simulink model "simulation_model_3"  (R2022b)
settings: Solver=ode3  StartTime=0.0  StopTime=Tsim  FixedStep=DTsim  RelTol=1e-3  EnableMultiTasking=on
values from neighbouring files (symbols this model uses):
  d1_step_final_value = 10    [simulation_script.m]
  d1_step_initial_value = 0    [simulation_script.m]
  d1_step_start = 5    [simulation_script.m]
  d1_step_stop = Tsim+1    (= 101)    [simulation_script.m]
  d2_step_final_value = 5    [simulation_script.m]
  d2_step_initial_value = 0    [simulation_script.m]
  d2_step_start = 10    [simulation_script.m]
  d2_step_stop = Tsim+1    (= 101)    [simulation_script.m]
  f = 0.1    [simulation_script.m]
  g = 9.81    [simulation_script.m]
  J = 0.2    [simulation_script.m]
  kd_gx = 2*omega*epsilon    (= 8)    [simulation_script.m]
  kd_gz = 2*omega*epsilon    (= 8)    [simulation_script.m]
  kp_gx = omega^2    (= 32.6530612245)    [simulation_script.m]
  kp_gz = omega^2    (= 32.6530612245)    [simulation_script.m]
  Lmax = 200    [simulation_script.m]
  Lmin = 0    [simulation_script.m]
  m = 10    [simulation_script.m]
  tau = 0.1    [simulation_script.m]
  Tmax = 0.035    [simulation_script.m]
  Tmin = -0.035    [simulation_script.m]
settings Model: Creator=mouyon  LastModifiedBy=Akash
settings SolverCC: AlgebraicLoopSolver=TrustRegion
settings DataIOCC: LimitDataPoints=on  SaveFormat=Array  SignalLoggingSaveFormat=ModelDataLogs  ReturnWorkspaceOutputs=off
settings OptimizationCC: ExpressionDepthLimit=2147483647  InitFltsAndDblsToZero=on  LifeSpan=inf
settings DebuggingCC: UnderspecifiedInitializationDetection=Classic  MergeDetectMultiDrivingBlocksExec=none  SolverPrmCheckMsg=warning  FcnCallInpInsideContextMsg=warning  UnconnectedInputMsg=warning  UnconnectedOutputMsg=warning  UnconnectedLineMsg=warning  AllowSymbolicDim=off  StateNameClashWarn=warning  SFUnexpectedBacktrackingDiag=warning  SFNoUnconditionalDefaultTransitionDiag=warning  SFExecutionAtInitializationDiag=none  SFMachineParentedDataDiag=warning  ArithmeticOperatorsInVariantConditions=warning
settings HardwareCC: ProdBitPerPointer=32  ProdBitPerSizeT=32  ProdBitPerPtrDiffT=32  ProdLargestAtomicFloat=None  ProdIntDivRoundTo=Undefined  ProdEndianess=Unspecified  ProdWordSize=32  ProdHWDeviceType=32-bit Generic
settings ModelReferenceCC: EnableRefExpFcnMdlSchedulingChecks=on  PropagateSignalLabelsOutOfModel=off
settings SFSimCC: SimUseLocalCustomCode=off  CustomCodeUndefinedFunction=UseInterfaceOnly
settings RTWCC: RTWUseLocalCustomCode=off
settings CodeAppCC: StateflowObjectComments=on
settings GRTTargetCC: TargetLangStandard=C89/C90 (ANSI)  CombineOutputUpdateFcns=off  GRTInterface=on
settings ConfigComp: CovMetricSettings=dw  CovSaveCumulativeToWorkspaceVar=on  CovSaveSingleToWorkspaceVar=on  CovExternalEMLEnable=off

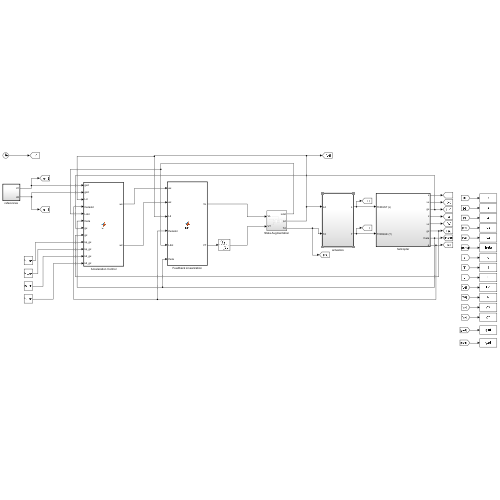
[thumbnail: Simulink's stored preview of the top-level diagram]
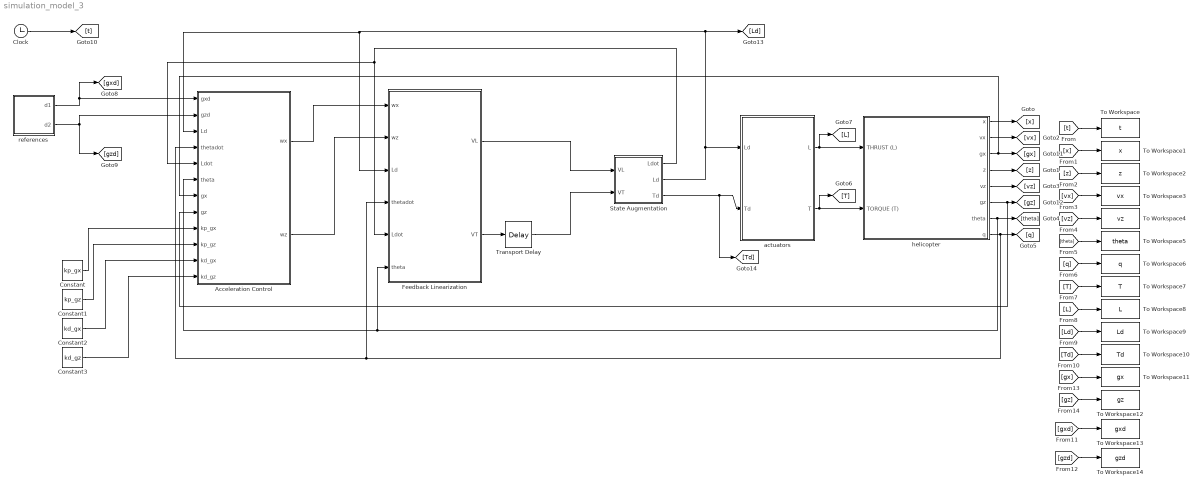
== system simulation_model_3 ==
  Acceleration Control : MATLAB Function  TreatAsAtomicUnit=on
  Clock : Clock
  Constant : Constant  Value=kp_gx
  Constant1 : Constant  Value=kp_gz
  Constant2 : Constant  Value=kd_gx
  Constant3 : Constant  Value=kd_gz
  Feedback Linearization : MATLAB Function  TreatAsAtomicUnit=on
  State Augmentation : Subsystem
  To Workspace : ToWorkspace  VariableName=t  SampleTime=-1
  To Workspace1 : ToWorkspace  VariableName=x  SampleTime=-1
  To Workspace10 : ToWorkspace  VariableName=Td  SampleTime=-1
  To Workspace11 : ToWorkspace  VariableName=gx  SampleTime=-1
  To Workspace12 : ToWorkspace  VariableName=gz  SampleTime=-1
  To Workspace13 : ToWorkspace  VariableName=gxd  SampleTime=-1
  To Workspace14 : ToWorkspace  VariableName=gzd  SampleTime=-1
  To Workspace2 : ToWorkspace  VariableName=z  SampleTime=-1
  To Workspace3 : ToWorkspace  VariableName=vx  SampleTime=-1
  To Workspace4 : ToWorkspace  VariableName=vz  SampleTime=-1
  To Workspace5 : ToWorkspace  VariableName=theta  SampleTime=-1
  To Workspace6 : ToWorkspace  VariableName=q  SampleTime=-1
  To Workspace7 : ToWorkspace  VariableName=T  SampleTime=-1
  To Workspace8 : ToWorkspace  VariableName=L  SampleTime=-1
  To Workspace9 : ToWorkspace  VariableName=Ld  SampleTime=-1
  Transport Delay : TransportDelay  DelayTime=0
  actuators : Subsystem  TreatAsAtomicUnit=on
  helicopter : Subsystem  TreatAsAtomicUnit=on
  references : Subsystem  TreatAsAtomicUnit=on
  wires:
  helicopter/1(x) -> [x]
  helicopter/5(vz) -> [vz]
  helicopter/7(theta) -> Feedback Linearization/6(theta), Acceleration Control/6(theta), [theta]
  helicopter/8(q) -> Acceleration Control/4(thetadot), Feedback Linearization/4(thetadot), [q]
  Clock/1 -> [t]
  [t] -> To Workspace/1
  [x] -> To Workspace1/1
  [z] -> To Workspace2/1
  [vx] -> To Workspace3/1
  [vz] -> To Workspace4/1
  [theta] -> To Workspace5/1
  [q] -> To Workspace6/1
  [T] -> To Workspace7/1
  [L] -> To Workspace8/1
  [Ld] -> To Workspace9/1
  [Td] -> To Workspace10/1
  helicopter/2(vx) -> [vx]
  helicopter/4(z) -> [z]
  helicopter/3(gx) -> Acceleration Control/7(gx), [gx]
  helicopter/6(gz) -> Acceleration Control/8(gz), [gz]
  [gx] -> To Workspace11/1
  [gz] -> To Workspace12/1
  actuators/1(L) -> helicopter/1(THRUST (L)), [L]
  actuators/2(T) -> helicopter/2(TORQUE (T)), [T]
  references/2(d2) -> [gzd], Acceleration Control/2(gzd)
  [gxd] -> To Workspace13/1
  [gzd] -> To Workspace14/1
  Feedback Linearization/2(VT) -> Transport Delay/1
  references/1(d1) -> [gxd], Acceleration Control/1(gxd)
  Acceleration Control/1(wx) -> Feedback Linearization/1(wx)
  Acceleration Control/2(wz) -> Feedback Linearization/2(wz)
  State Augmentation/1(Ldot) -> Feedback Linearization/5(Ldot), Acceleration Control/5(Ldot)
  State Augmentation/2(Ld) -> Acceleration Control/3(Ld), Feedback Linearization/3(Ld), [Ld], actuators/1(Ld)
  State Augmentation/3(Td) -> [Td], actuators/2(Td)
  Feedback Linearization/1(VL) -> State Augmentation/1(VL)
  Transport Delay/1 -> State Augmentation/2(VT)
  Constant/1 -> Acceleration Control/9(kp_gx)
  Constant1/1 -> Acceleration Control/10(kp_gz)
  Constant3/1 -> Acceleration Control/12(kd_gz)
  Constant2/1 -> Acceleration Control/11(kd_gx)

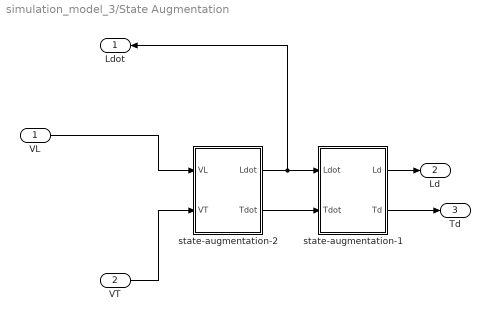
== system simulation_model_3/State Augmentation ==
  VL : Inport
  VT : Inport  Port=2
  state-augmentation-1 : Subsystem  TreatAsAtomicUnit=on
  state-augmentation-2 : Subsystem  TreatAsAtomicUnit=on
  Ldot : Outport
  Ld : Outport  Port=2
  Td : Outport  Port=3
  wires:
  state-augmentation-2/2(Tdot) -> state-augmentation-1/2(Tdot)
  state-augmentation-2/1(Ldot) -> Ldot/1, state-augmentation-1/1(Ldot)
  state-augmentation-1/1(Ld) -> Ld/1
  state-augmentation-1/2(Td) -> Td/1
  VL/1 -> state-augmentation-2/1(VL)
  VT/1 -> state-augmentation-2/2(VT)

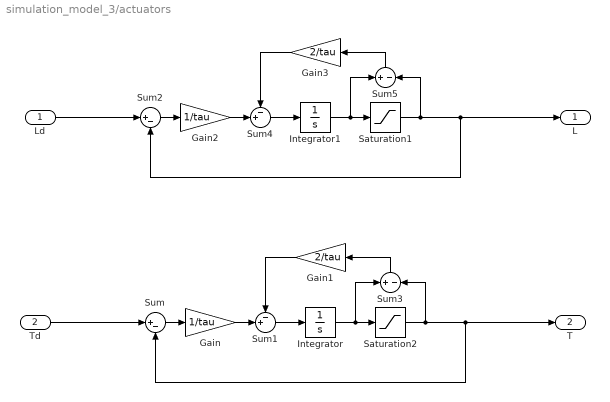
== system simulation_model_3/actuators ==
  Ld : Inport
  Td : Inport  Port=2
  Gain : Gain  Gain=1/tau
  Gain1 : Gain  Gain=2/tau
  Gain2 : Gain  Gain=1/tau
  Gain3 : Gain  Gain=2/tau
  Integrator : Integrator
  Integrator1 : Integrator  InitialCondition=m*g
  Saturation1 : Saturate  UpperLimit=Lmax  LowerLimit=Lmin
  Saturation2 : Saturate  UpperLimit=Tmax  LowerLimit=Tmin
  Sum : Sum  Inputs=|+-
  Sum1 : Sum  Inputs=-+|
  Sum2 : Sum  Inputs=|+-
  Sum3 : Sum  Inputs=+|-  SaturateOnIntegerOverflow=on
  Sum4 : Sum  Inputs=-+|
  Sum5 : Sum  Inputs=+|-  SaturateOnIntegerOverflow=on
  L : Outport
  T : Outport  Port=2
  wires:
  Integrator/1 -> Sum3/1, Saturation2/1
  Sum/1 -> Gain/1
  Td/1 -> Sum/1
  Sum3/1 -> Gain1/1
  Gain/1 -> Sum1/2
  Sum1/1 -> Integrator/1
  Integrator1/1 -> Saturation1/1, Sum5/1
  Sum2/1 -> Gain2/1
  Ld/1 -> Sum2/1
  Saturation1/1 -> Sum2/2, L/1, Sum5/2
  Sum5/1 -> Gain3/1
  Gain2/1 -> Sum4/2
  Sum4/1 -> Integrator1/1
  Gain3/1 -> Sum4/1
  Gain1/1 -> Sum1/1
  Saturation2/1 -> Sum/2, T/1, Sum3/2

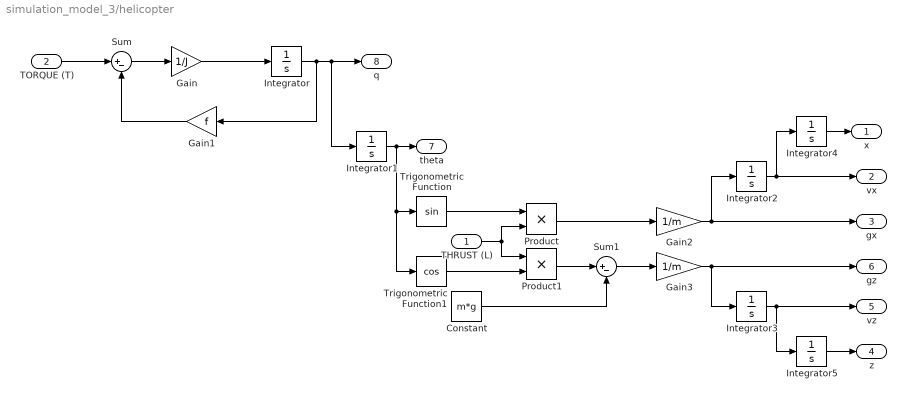
== system simulation_model_3/helicopter ==
  THRUST (L) : Inport
  TORQUE (T) : Inport  Port=2
  Constant : Constant  Value=m*g
  Gain : Gain  Gain=1/J
  Gain1 : Gain  Gain=f
  Gain2 : Gain  Gain=1/m
  Gain3 : Gain  Gain=1/m
  Integrator{,1..5} (6 alike) : Integrator
  Product : Product  RndMeth=Zero
  Product1 : Product  RndMeth=Zero
  Sum : Sum  Inputs=|+-
  Sum1 : Sum  Inputs=|+-
  Trigonometric Function : Trigonometry
  Trigonometric Function1 : Trigonometry  Operator=cos
  x : Outport
  vx : Outport  Port=2
  gx : Outport  Port=3
  z : Outport  Port=4
  vz : Outport  Port=5
  gz : Outport  Port=6
  theta : Outport  Port=7
  q : Outport  Port=8
  wires:
  Integrator/1 -> Gain1/1, q/1, Integrator1/1
  Gain/1 -> Integrator/1
  Gain1/1 -> Sum/2
  Sum/1 -> Gain/1
  TORQUE (T)/1 -> Sum/1
  Integrator1/1 -> theta/1, Trigonometric Function/1, Trigonometric Function1/1
  Trigonometric Function/1 -> Product/1
  THRUST (L)/1 -> Product/2, Product1/1
  Trigonometric Function1/1 -> Product1/2
  Product/1 -> Gain2/1
  Product1/1 -> Sum1/1
  Constant/1 -> Sum1/2
  Gain3/1 -> gz/1, Integrator3/1
  Sum1/1 -> Gain3/1
  Integrator2/1 -> vx/1, Integrator4/1
  Integrator3/1 -> vz/1, Integrator5/1
  Integrator4/1 -> x/1
  Integrator5/1 -> z/1
  Gain2/1 -> gx/1, Integrator2/1

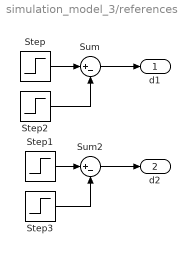
== system simulation_model_3/references ==
  Step : Step  Time=d1_step_start  Before=d1_step_initial_value  After=d1_step_final_value  SampleTime=0
  Step1 : Step  Time=d2_step_start  Before=d2_step_initial_value  After=d2_step_final_value  SampleTime=0
  Step2 : Step  Time=d1_step_stop  After=d1_step_final_value  SampleTime=0
  Step3 : Step  Time=d2_step_stop  After=d2_step_final_value  SampleTime=0
  Sum : Sum  Inputs=|+-
  Sum2 : Sum  Inputs=|+-
  d1 : Outport
  d2 : Outport  Port=2
  wires:
  Step/1 -> Sum/1
  Step2/1 -> Sum/2
  Step1/1 -> Sum2/1
  Sum/1 -> d1/1
  Sum2/1 -> d2/1
  Step3/1 -> Sum2/2

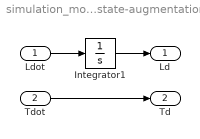
== system simulation_model_3/State Augmentation/state-augmentation-1 ==
  Ldot : Inport
  Tdot : Inport  Port=2
  Integrator1 : Integrator  InitialCondition=m*g
  Ld : Outport
  Td : Outport  Port=2
  wires:
  Integrator1/1 -> Ld/1
  Ldot/1 -> Integrator1/1
  Tdot/1 -> Td/1

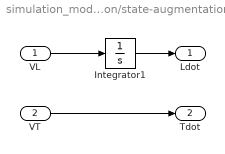
== system simulation_model_3/State Augmentation/state-augmentation-2 ==
  VL : Inport
  VT : Inport  Port=2
  Integrator1 : Integrator
  Ldot : Outport
  Tdot : Outport  Port=2
  wires:
  Integrator1/1 -> Ldot/1
  VL/1 -> Integrator1/1
  VT/1 -> Tdot/1

== matlab function simulation_model_3/Feedback Linearization ==
  data: wx input; VL output; wz input; VT output; Ld input; thetadot input; Ldot input; theta input
function [VL,VT] = fcn(wx, wz, Ld, thetadot, Ldot, theta)

m = 10;
J = 0.2;
f = 0.1;

A1 = [Ld*thetadot^2;
(thetadot*(Ld*f - 2*J*Ldot))/Ld];

A2 = [m*sin(theta)        m*cos(theta);
(J*m*cos(theta))/Ld -(J*m*sin(theta))/Ld];

Answer = A1 + A2*[wx;wz];
VL = Answer(1);
VT = Answer(2);
end

== matlab function simulation_model_3/Acceleration Control ==
  data: gxd input; wx output; gzd input; wz output; Ld input; thetadot input; Ldot input; theta input; gx input; gz input; kp_gx input; kp_gz input; kd_gx input; kd_gz input
function [wx,wz]  = fcn(gxd, gzd, Ld, thetadot, Ldot, theta, gx, gz, kp_gx, kp_gz, kd_gx, kd_gz)

m = 10;
%alpha1 = 8.792;
%alpha2 = 39.4384;
gxdot = (Ld*cos(theta)*thetadot/m + sin(theta)*Ldot/m);
gzdot = (-Ld*sin(theta)*thetadot/m + cos(theta)*Ldot/m);

wx = -kd_gx*gxdot - kp_gx*gx + kp_gx*gxd;
wz = -kd_gz*gzdot - kp_gz*gz + kp_gz*gzd;

end
